simulink model "Sub3_2023"  (R2023b)
settings: Solver=FixedStepDiscrete  StartTime=0.0  StopTime=4.5  FixedStep=75e-6  RelTol=1e-3  EnableMultiTasking=on
undefined symbols (not defined in the file or in its folder): D1, D11, Delta
libraries: spsSeriesRLCBranchLib x41, spsLoadFlowBusLib x29, spsDistributedParametersLineLib x19, spsThreePhaseSeriesRLCLoadLib x15, spsThreePhaseTransformerTwoWindingsLib x13, spsThreePhaseParallelRLCLoadLib x11, spsThreePhaseVIMeasurementLib x11, spsSynchronousMachinepuStandardLib x7, spsExcitationSystemLib x7, spsHydraulicTurbineandGovernorLib x7, spsGenericPowerSystemStabilizerLib x7, spsMultiBandPowerSystemStabilizerLib x7
(part 1 of 5)
settings Model: Creator=The MathWorks, Inc.  LastModifiedBy=dilu2
settings SolverCC: AlgebraicLoopSolver=TrustRegion
settings DataIOCC: SaveFormat=StructureWithTime  SaveOutput=off  SignalLogging=off  DSMLogging=off  SaveTime=off  ReturnWorkspaceOutputs=off
settings OptimizationCC: ExpressionDepthLimit=2147483647  LifeSpan=inf
settings DebuggingCC: UnderspecifiedInitializationDetection=Classic  MergeDetectMultiDrivingBlocksExec=none  SolverPrmCheckMsg=warning  FcnCallInpInsideContextMsg=warning  UnconnectedInputMsg=warning  UnconnectedOutputMsg=warning  UnconnectedLineMsg=warning  StateNameClashWarn=warning  SFUnexpectedBacktrackingDiag=warning  SFNoUnconditionalDefaultTransitionDiag=warning  SFExecutionAtInitializationDiag=none  ArithmeticOperatorsInVariantConditions=warning
settings HardwareCC: ProdBitPerPointer=32  ProdBitPerSizeT=32  ProdBitPerPtrDiffT=32  ProdLargestAtomicFloat=None  ProdIntDivRoundTo=Undefined  ProdEndianess=Unspecified  ProdWordSize=32  ProdHWDeviceType=32-bit Generic
settings ModelReferenceCC: EnableRefExpFcnMdlSchedulingChecks=on  PropagateSignalLabelsOutOfModel=off
settings SFSimCC: SimUseLocalCustomCode=off  CustomCodeUndefinedFunction=UseInterfaceOnly
settings RTWCC: RTWUseLocalCustomCode=off
settings CodeAppCC: StateflowObjectComments=on
settings GRTTargetCC: TargetLangStandard=C89/C90 (ANSI)  CombineOutputUpdateFcns=off  GRTInterface=on
settings ConfigComp: CovMetricSettings=dw  CovSaveCumulativeToWorkspaceVar=on  CovSaveSingleToWorkspaceVar=on  CovExternalEMLEnable=off  CovSFcnEnable=off
settings SimscapeCC: SimscapeNormalizeSystem=off

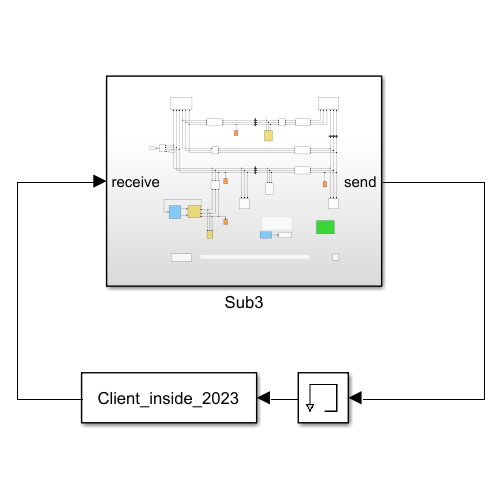
[thumbnail: Simulink's stored preview of the top-level diagram]
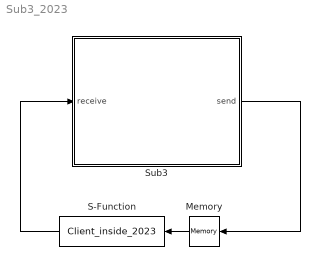
== system Sub3_2023 ==
  Memory : Memory
  S-Function : S-Function  FunctionName=Client_inside_2023  SFunctionDeploymentMode=off  EnableBusSupport=off
  Sub3 : Subsystem
  wires:
  Memory/1 -> S-Function/1
  S-Function/1 -> Sub3/1(receive)
  Sub3/1(send) -> Memory/1

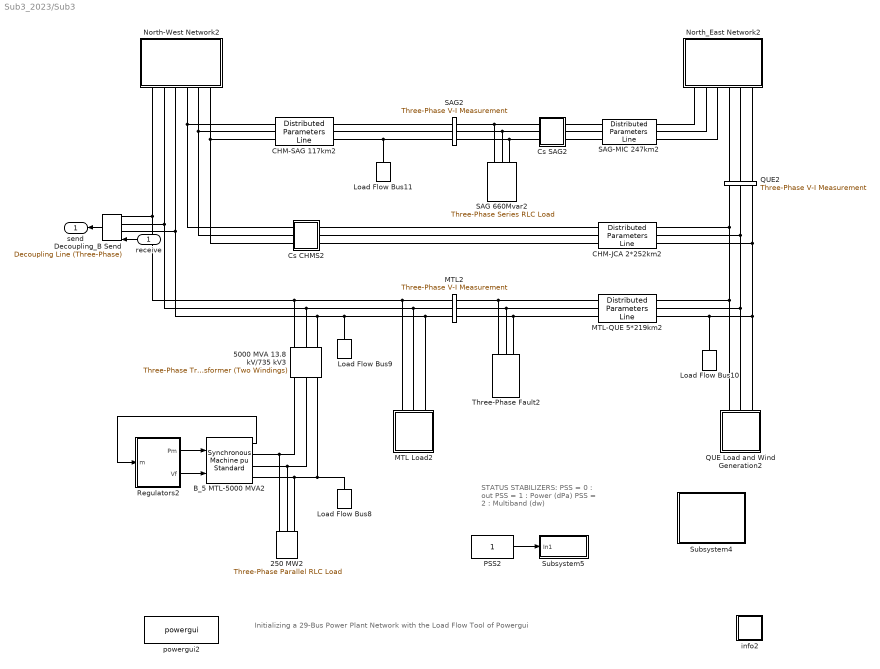
== system Sub3_2023/Sub3 ==
  note: Initializing a 29-Bus Power Plant Network with the Load Flow Tool of Powergui
  note: STATUS STABILIZERS:
      | PSS = 0 :  out
      | PSS = 1 :  Power (dPa)
      | PSS = 2 :  Multiband (dw)
  receive : Inport
  250 MW2 : spsThreePhaseParallelRLCLoadLib/Three-Phase Parallel RLC Load  LConnTagsString=A|B|C  Configuration=Y (grounded)  NominalVoltage=(13800)*1  Vabc=[1e3 1e3 1e3]  Vabcp=[1e3 1e3 1e3]  NominalFrequency=60  UnbalancedPower=off  ActivePower=250000000  InductivePower=0  CapacitivePower=0  Pabc=[10e3 9e3 11e3]  QLabc=[100 90 110]  QCabc=[100 90 110]  Pabcp=[10e3 9e3 11e3]  QLabcp=[100 90 110]  QCabcp=[100 90 110]  Measurements=None  LoadType=constant PQ
  5000 MVA 13.8 kV/735 kV3 : spsThreePhaseTransformerTwoWindingsLib/Three-Phase Transformer (Two Windings)  Winding1Connection=Delta (D1)  Winding2Connection=Yg  CoreType=Three single-phase transformers  SetSaturation=off  Hysteresis=off  DataFile='basic_model'  SetInitialFlux=off  Measurements=None  UNITS=pu  NominalPower=[ 5000e6 60 ]  Winding1="[ 13.8e3 0.002  0.0]"  Winding2=[ 735e3 0.002 0.12]  Rm=500  Lm=500  L0=0.5  Saturation="[ 0,0  ;  0.005,1.2  ;  1.0,1.4 ]"  InitialFluxes=[ 0.8 , -0.8 , 0.7 ]  BreakLoop=off  DiscreteSolver=Trapezoidal iterative  DataType=off  TransfoNumber=0
  B_5 MTL-5000 MVA2 : spsSynchronousMachinepuStandardLib/Synchronous Machine pu Standard  PresetModel=No  MechanicalLoad=Mechanical power Pm  ShowDetailedParameters=on  RotorType=Salient-pole  Units=per unit standard parameters  MeasurementBus=off  NominalParameters="[5000E6  13800   60 ]"  Reactances1=[ 31 32 33 34 35 36 37 ]  Reactances2=[ 1.305, 0.296, 0.252, 0.474, 0.243, 0.18 ]  dAxisTimeConstants=Short-circuit  qAxisTimeConstants=Open-circuit  TimeConstants1=[]  TimeConstants2=[]  TimeConstants3=[]  TimeConstants4=[]  TimeConstants5=[ 1.01, 0.053, 0.1 ]  TimeConstants6=[]  TimeConstants7=[]  TimeConstants8=[]  StatorResistance=2.8544e-3  Mechanical="[ 3.7 0  32]"  PolePairs=32  InitialConditions=[0 -113.876 0.904539 0.904539 0.904539 -42.1129 -162.113 77.8871 1.28555]  SetSaturation=off  Saturation=[0.6404,0.7127,0.8441,0.9214,0.9956,1.082,1.19,1.316,1.457;0.7,0.7698,0.8872,0.9466,0.9969,1.046,1.1,1.151,1.201]  LoadFlowParameters=[1 4000000000 0 0 0]  TsPowergui=0  TsBlock=-1  IterativeModel=Trapezoidal non iterative  IterativeDiscreteModel=Trapezoidal non iterative  BusType=PV  Pref=4500000000  Qref=0  Qmin=-Inf  Qmax=Inf  PLF=0  QLF=0
  CHM-JCA 2*252km2 : spsDistributedParametersLineLib/Distributed Parameters Line  Phases=3  Length=252  Frequency=60  Resistance="[0.01273  0.3864]/2"  Inductance="[0.9337e-3  4.1264e-3]/2"  Capacitance=[12.74e-9 7.751e-9]*2  x1=[-0.0015 2.14788825310089e-08 -52695.4931206876 -817990.561269633;-0.001425 2.14931441848027e-08 -29549.3766894674 -819153.330536621;-0.00135 2.14902245479913e-08 -6379.63893864228 -819661.281164644;-0.001275 2.14701259544877e-08 16795.1985979387 -819514.007105742;-0.0012 2.14328644708e-08 39956.6103097356 -818711.626088545;-0.001125 2.13784698831882e-08 63086.0813186075 -817254.77952416;-0.00105 2.13069856738533e-08 86165.1222793228 -815144.631993441;-0.000975 2.12184689861786e-08 109175.284159659 -812382.870316038;-0.0009 2.11129905790498e-08 132098.172988275 -808971.702201979;-0.000825 2.09906347702916e-08 154915.464558574 -804913.854486862;-0.00075 2.08514993692656e-08 177608.919076792 -800212.570952063;-0.000675 2.06956955986824e-08 200160.395742607 -794871.609731707;-0.0006 2.05233480056924e-08 222551.867250622 -788895.240308476;-0.000525 2.03345943623244e-08 244765.434201114 -782288.240100644;-0.00045 2.01295855553529e-08 266783.339408543 -775055.890643087;-0.000375 1.99084854656814e-08 288587.982096371 -767203.973365303;-0.0003 1.96714708373387e-08 310161.931966855 -758738.764969824;-0.000225 1.94187311361923e-08 331487.943134562 -749667.032414722;-0.00015 1.91504683984921e-08 352548.967912462 -739996.027504197;-7.5e-05 1.88668970693661e-08 373328.170439593 -729733.481091605]  x2=[-0.0015 1.43547805261935e-08 -269861.286315616 -765335.489949611;-0.001425 1.43176491173949e-08 -248116.944399225 -772658.724453944;-0.00135 1.42690723989592e-08 -226174.261593797 -779364.307396023;-0.001275 1.4209089202372e-08 -204050.778544234 -785446.878435444;-0.0012 1.41377474772827e-08 -181764.180424385 -790901.575257983;-0.001125 1.40551042531748e-08 -159332.282799789 -795724.037462462;-0.00105 1.39612255937773e-08 -136773.017386189 -799910.410046378;-0.000975 1.3856186544254e-08 -114104.417715188 -803457.346487544;-0.0009 1.3740071071214e-08 -91344.604718521 -806362.011419237;-0.000825 1.36129719955899e-08 -68511.7722424616 -808622.082896754;-0.00075 1.34749909184379e-08 -45624.1725039369 -810235.754253535;-0.000675 1.33262381397199e-08 -22700.1014999858 -811201.73554539;-0.0006 1.31668325701314e-08 242.115617781237 -811519.254581652;-0.000525 1.29969016360456e-08 23184.1391920279 -811188.057542463;-0.00045 1.28165811776512e-08 46107.6297201337 -810208.409181668;-0.000375 1.26260153403637e-08 68994.2625145116 -808581.092615177;-0.0003 1.24253564595976e-08 91825.742351083 -806307.408694955;-0.000225 1.2214764938992e-08 114583.8180942 -803389.17496914;-0.00015 1.19944091221863e-08 137250.297286324 -799828.72422912;-7.5e-05 1.1764465158249e-08 159807.060690796 -795628.902644742]  x3=[-0.0015 5.32909393588854e-11 -353.825063947876 -933.331217282833;-0.001425 5.27444551797059e-11 -327.297425889231 -942.960561676809;-0.00135 5.2155807890073e-11 -300.508151276149 -951.836117825561;-0.001275 5.15254680456233e-11 -273.478655044866 -959.950790745304;-0.0012 5.08539395303841e-11 -246.230544161103 -967.298093690665;-0.001125 5.01417591539757e-11 -218.785600347792 -973.872153340087;-0.00105 4.93894962224943e-11 -191.165762673095 -979.667714490872;-0.000975 4.85977520834172e-11 -163.393110012651 -984.680144260112;-0.0009 4.77671596448951e-11 -135.489843400061 -988.905435788142;-0.000825 4.6898382869815e-11 -107.478268279722 -992.340211441564;-0.00075 4.59921162450381e-11 -79.3807766761923 -994.981725513273;-0.000675 4.50490842262379e-11 -51.2198292943543 -996.827866417338;-0.0006 4.40700406587813e-11 -23.0179375646682 -997.877158376967;-0.000525 4.30557681751163e-11 5.20235435212098 -998.128762604222;-0.00045 4.20070775691475e-11 33.4184875864397 -997.582477970533;-0.000375 4.09248071480997e-11 61.6079065931019 -996.238741167479;-0.0003 3.98098220623883e-11 89.7480771818661 -994.098626357699;-0.000225 3.8663013614031e-11 117.816504530923 -991.163844316227;-0.00015 3.74852985441545e-11 145.79075116891 -987.436741062925;-7.5e-05 3.62776183001661e-11 173.648454911087 -982.920295987105]  x4=[-0.0015 3.56468616185308e-11 -3930.11452440296 -10267.8671256367;-0.001425 3.68276356651575e-11 -3638.26562484361 -10374.8700196272;-0.00135 3.79789702633153e-11 -3343.50835141109 -10473.5794012647;-0.001275 3.90999450537422e-11 -3046.07832855985 -10563.9163637801;-0.0012 4.01896639463424e-11 -2746.21331729932 -10645.8086931875;-0.001125 4.12472558365064e-11 -2444.15302513141 -10719.190926012;-0.00105 4.22718753014589e-11 -2140.138914432 -10784.0044016194;-0.000975 4.32627032760768e-11 -1834.41400942963 -10840.1973091089;-0.0009 4.42189477076373e-11 -1527.22270193559 -10887.72472873;-0.000825 4.51398441889729e-11 -1218.81055598091 -10926.5486677908;-0.00075 4.60246565695266e-11 -909.424111516214 -10956.6380910284;-0.000675 4.68726775438196e-11 -599.310687331423 -10977.9689454182;-0.0006 4.768322921686e-11 -288.718183352941 -10990.5241794015;-0.000525 4.84556636460423e-11 22.1051175237762 -10994.2937565166;-0.00045 4.91893633591025e-11 332.910747907765 -10989.274663421;-0.000375 4.98837418477159e-11 643.450254533582 -10975.470912301;-0.0003 5.05382440363431e-11 953.475396871044 -10952.893537664;-0.000225 5.11523467259487e-11 1262.73834556491 -10921.5605875179;-0.00015 5.17255590122387e-11 1570.99188054588 -10881.4971089437;-7.5e-05 5.2257422678082e-11 1877.98958865452 -10832.735128073]  x5=0.00142516474882927  V1=ones(3,3)  V2=ones(3,3)  I1=ones(3,3)  I2=ones(3,3)  nHarmo=1  Measurements=None  Decoupling=on  VsMag0=[669271.096488228 669270.652926469 669270.90062472]  VrMag0=[662602.894278608 662603.037872478 662602.726163221]  VsAngle0=[-1.28592943401852 -121.285926872022 118.714104732553]  VrAngle0=[-17.0228975012821 -137.022921456009 102.977079768198]  IsMag0=[819.838115462759 819.831333521817 819.822841412156]  IrMag0=[9030.15416595123 9030.15837069581 9030.1660687479]  IsAngle0=[-18.3607604375241 -138.36171938416 101.639170566658]  IrAngle0=[-18.5448447465942 -138.544772943748 101.455168050306]
      settings: AttributesFormatString=\n  LibrarySourceBlock=sps_lib/Power Grid Elements/Distributed Parameters Line
  CHM-SAG 117km2 : spsDistributedParametersLineLib/Distributed Parameters Line  Phases=3  Length=117  Frequency=60  Resistance="[0.01273  0.3864]"  Inductance="[0.9337e-3  4.1264e-3]"  Capacitance=[12.74e-9 7.751e-9]  x1=[-0.000675 1.98658437347204e-08 120099.384212573 -820048.654169142;-0.0006 1.97055789462812e-08 143234.627617142 -816325.600270959;-0.000525 1.95295618195378e-08 166255.371451958 -811949.988178119;-0.00045 1.93379330598881e-08 189143.213286628 -806925.315687981;-0.000375 1.91308458524307e-08 211879.856930585 -801255.599446853;-0.0003 1.89084657395106e-08 234447.127058782 -794945.37173915;-0.000225 1.86709704883876e-08 256826.983740769 -787999.67686435;-0.00015 1.84185499491316e-08 279001.536861539 -780424.067104664;-7.5e-05 1.81514059028595e-08 300953.060422608 -772224.598286623]  x2=[-0.000675 1.36464150047778e-08 166130.546631654 -803426.098272825;-0.0006 1.3510914913813e-08 188777.466023371 -798408.377649309;-0.000525 1.33646144041902e-08 211273.479597141 -792752.421584757;-0.00045 1.3207630426298e-08 233600.604383914 -786462.751363909;-0.000375 1.30400884707266e-08 255740.992421751 -779544.394852905;-0.0003 1.28621224679518e-08 277676.945023215 -772002.882480085;-0.000225 1.26738746812731e-08 299390.926923427 -763844.24281505;-0.00015 1.2475495593091e-08 320865.580297491 -755074.997749517;-7.5e-05 1.22671437846133e-08 342083.738636073 -745702.157283819]  x3=[-0.000675 1.56671377221203e-11 655.342290944049 -4153.32595111528;-0.0006 1.47007289951298e-11 772.497655199839 -4133.1388980955;-0.000525 1.37225687303092e-11 889.035496649674 -4109.64787707972;-0.00045 1.2733438854008e-11 1004.86265672619 -4082.87166643073;-0.000375 1.1734130061515e-11 1119.88654496983 -4052.83167064162;-0.0003 1.07254411849891e-11 1234.01521304425 -4019.55190322541;-0.000225 9.70817855488465e-12 1347.15742823844 -3983.05896751897;-0.00015 8.68315535538353e-12 1459.2227463967 -3943.38203541674;-7.5e-05 7.65119097434806e-12 1570.12158421834 -3900.55282405116]  x4=[-0.000675 2.87955679117454e-11 -58.179032260622 -1899.1904056796;-0.0006 2.95286509391463e-11 -4.4649544291961 -1900.07615984008;-0.000525 3.02381292147899e-11 49.2526926184844 -1899.44302219052;-0.00045 3.0923435592598e-11 102.930967817277 -1897.29149885148;-0.000375 3.15840222491379e-11 156.526961575294 -1893.62330971778;-0.0003 3.22193611215436e-11 209.99783007517 -1888.44138708371;-0.000225 3.28289443296414e-11 263.300829522758 -1881.74987329893;-0.00015 3.34122845819419e-11 316.393350315863 -1873.55411745716;-7.5e-05 3.39689155651726e-11 369.232951105707 -1863.86067112024]  x5=0.000661683633385019  V1=ones(3,3)  V2=ones(3,3)  I1=ones(3,3)  I2=ones(3,3)  nHarmo=1  Measurements=None  Decoupling=on  VsMag0=[676709.77841619 676709.532429466 676709.555770503]  VrMag0=[669872.175479888 669872.308250308 669872.011404575]  VsAngle0=[-7.08802978836752 -127.088039531023 112.911983377236]  VrAngle0=[-3.73716141990226 -123.737184181178 116.262817364722]  IsMag0=[3442.59994794228 3442.59576511442 3442.58917191232]  IrMag0=[1555.67453781717 1555.67655932668 1555.6835352225]  IsAngle0=[-6.45330477220459 -126.453471672169 113.546672066862]  IrAngle0=[-17.1748303043255 -137.174490649355 102.825275045827]
      settings: AttributesFormatString=\n  LibrarySourceBlock=sps_lib/Power Grid Elements/Distributed Parameters Line
  Cs CHMS2 : Subsystem  mask{Xc=33/2}
      mask prompts: Xc "Condensator Reactance at  60Hz  (ohm):"
      mask help: Series Compensation
      mask init:
      | Cs=1/Xc/(2*pi*60);
      mask Display: disp('Cs')
  Cs SAG2 : Subsystem  mask{Xc=22}
      mask prompts: Xc "Condensator Reactance at  60Hz  (ohm):"
      mask help: Series Compensation
      mask init:
      | Cs=1/Xc/(2*pi*60);
      mask Display: disp('Cs')
  Decoupling_B Send : spsDecouplingLineThreePhaseLib/Decoupling Line (Three-Phase)  Length=252  Frequency=60  Resistance="[0.01273  0.3864]/2"  Inductance="[0.9337e-3  4.1264e-3]/2"  Capacitance=[12.74e-9 7.751e-9]*2  VsMag0=[645716.873803131 645717.117585077 645717.103800347]  VsAngle0=[95.8608940156624 -144.139117060793 -24.1390927893461]  IhsMag0=[6636.13895491375 6636.14647590145 6636.14203567859]  IhsAngle0=[111.871942870248 -128.128050353118 -8.12799750568943]  ShowPorts=on  ConnectorID=T42_4043_2846767750151_S
      settings: LibrarySourceBlock=|
      | sps_lib/Power Grid Elements/Decoupling Line
      | (Three-Phase)
  Load Flow Bus10 : spsLoadFlowBusLib/Load Flow Bus  LConnTagsString=a  Phases=single  Connectors=on one side  ID=QUE7  Vbase=735e3  Vref=1  Vangle=0  VLF=1.023  VLFb=1  VLFc=1  angleLF=-14.99  angleLFb=0  angleLFc=0
      settings: AttributesFormatString=%<ID>\n%<Vbase>V\n%<VLF>pu\n%<angleLF>deg.
  Load Flow Bus11 : spsLoadFlowBusLib/Load Flow Bus  LConnTagsString=a  Phases=single  Connectors=on one side  ID=SAG7  Vbase=735e3  Vref=1  Vangle=0  VLF=1.036  VLFb=1  VLFc=1  angleLF=-0.1653  angleLFb=0  angleLFc=0
      settings: AttributesFormatString=%<ID>\n%<Vbase>V\n%<VLF>pu\n%<angleLF>deg.
  Load Flow Bus8 : spsLoadFlowBusLib/Load Flow Bus  LConnTagsString=a  Phases=single  Connectors=on one side  ID=MTL_13.8  Vbase=13.8e3  Vref=1  Vangle=0  VLF=1  VLFb=1  VLFc=1  angleLF=-47.86  angleLFb=0  angleLFc=0
      settings: AttributesFormatString=%<ID>\n%<Vbase>V\n%<VLF>pu\n%<angleLF>deg.
  Load Flow Bus9 : spsLoadFlowBusLib/Load Flow Bus  LConnTagsString=a  Phases=single  Connectors=on one side  ID=MTL7  Vbase=735e3  Vref=1  Vangle=0  VLF=1.013  VLFb=1  VLFc=1  angleLF=-23.64  angleLFb=0  angleLFc=0
      settings: AttributesFormatString=%<ID>\n%<Vbase>V\n%<VLF>pu\n%<angleLF>deg.
  MTL Load2 : Subsystem
  MTL-QUE 5*219km2 : spsDistributedParametersLineLib/Distributed Parameters Line  Phases=3  Length=219  Frequency=60  Resistance="[0.01273  0.3864]/5"  Inductance="[0.9337e-3  4.1264e-3]/5"  Capacitance=[12.74e-9 7.751e-9]*5  x1=[-0.001275 8.97642211389418e-08 0 0;-0.0012 8.97304952684457e-08 0 0;-0.001125 8.96250402129547e-08 0 0;-0.00105 8.94479402716265e-08 0 0;-0.000975 8.91993370154446e-08 0 0;-0.0009 8.88794291740481e-08 0 0;-0.000825 8.84884724768708e-08 -163872.459638605 -773673.870997315;-0.00075 8.80267794487145e-08 -141934.751428708 -777997.40505494;-0.000675 8.74947191599218e-08 -119883.582750192 -781699.019890724;-0.0006 8.68927169313467e-08 -97736.5809699071 -784775.756490403;-0.000525 8.62212539943599e-08 -75511.4500622143 -787225.155357816;-0.00045 8.54808671061594e-08 -53225.9564567056 -789045.258480985;-0.000375 8.46721481206953e-08 -30897.9148359899 -790234.610897321;-0.0003 8.37957435155509e-08 -8545.17389490828 -790792.261856701;-0.000225 8.28523538751581e-08 13814.3979274394 -790717.765581479;-0.00015 8.18427333307609e-08 36162.9267314513 -790011.18162284;-7.5e-05 8.0767688957575e-08 58482.5474451453 -788673.074813188]  x2=[-0.001275 1.4209089202372e-08 0 0;-0.0012 1.41377474772827e-08 0 0;-0.001125 1.40551042531748e-08 0 0;-0.00105 1.39612255937773e-08 0 0;-0.000975 1.3856186544254e-08 0 0;-0.0009 1.3740071071214e-08 0 0;-0.000825 1.36129719955899e-08 -68511.7722424616 -808622.082896754;-0.00075 1.34749909184379e-08 -45624.1725039369 -810235.754253535;-0.000675 1.33262381397199e-08 -22700.1014999858 -811201.73554539;-0.0006 1.31668325701314e-08 242.115617781237 -811519.254581652;-0.000525 1.29969016360456e-08 23184.1391920279 -811188.057542463;-0.00045 1.28165811776512e-08 46107.6297201337 -810208.409181668;-0.000375 1.26260153403637e-08 68994.2625145116 -808581.092615177;-0.0003 1.24253564595976e-08 91825.742351083 -806307.408694955;-0.000225 1.2214764938992e-08 114583.8180942 -803389.17496914;-0.00015 1.19944091221863e-08 137250.297286324 -799828.72422912;-7.5e-05 1.1764465158249e-08 159807.060690796 -795628.902644742]  x3=[-0.001275 3.55264360188674e-10 0 0;-0.0012 3.29669675506793e-10 0 0;-0.001125 3.03811457930428e-10 0 0;-0.00105 2.77710378123064e-10 0 0;-0.000975 2.5138730088854e-10 0 0;-0.0009 2.2486326849204e-10 0 0;-0.000825 1.98159483839231e-10 -7102.47823834771 -20057.5471743782;-0.00075 1.71297293526982e-10 -6532.60058481189 -20250.3213202449;-0.000675 1.44298170779225e-10 -5957.5008703207 -20426.9076690885;-0.0006 1.17183698281583e-10 -5377.63882078661 -20587.1650604835;-0.000525 8.99755509285052e-11 -4793.47796905981 -20730.9653871235;-0.00045 6.26954784966872e-11 -4205.48528438722 -20858.1936972273;-0.000375 3.53652882586321e-11 -3614.13079912437 -20968.7482864307;-0.0003 8.00682755025e-12 -3019.88723299875 -21062.5407790865;-0.000225 -1.93580336935672e-11 -2423.22961522491 -21139.4961989112;-0.00015 -4.67074204214376e-11 -1824.6349047733 -21199.5530289196;-7.5e-05 -7.40194699520705e-11 -1224.58160909667 -21242.6632606007]  x4=[-0.001275 2.99597844132757e-10 0 0;-0.0012 3.28836590243948e-10 0 0;-0.001125 3.57812469416266e-10 0 0;-0.00105 3.86502318775247e-10 0 0;-0.000975 4.14883204094284e-10 0 0;-0.0009 4.42932438127893e-10 0 0;-0.000825 4.70627598747556e-10 -1323.85659522413 -8328.03394763917;-0.00075 4.97946546865624e-10 -1087.88942341492 -8362.13156092163;-0.000675 5.24867444132966e-10 -851.052609445902 -8389.54461417919;-0.0006 5.51368770396209e-10 -613.535477042433 -8410.25119383652;-0.000525 5.77429340900622e-10 -375.527893766024 -8424.23474737065;-0.00045 6.03028323224884e-10 -137.220119237107 -8431.48409654284;-0.000375 6.28145253934203e-10 101.197346955589 -8431.9934463343;-0.0003 6.52760054938472e-10 339.5339175375 -8425.76238957858;-0.000225 6.76853049542387e-10 577.599069900775 -8412.79590728711;-0.00015 7.00404978174696e-10 815.202498405133 -8393.10436466746;-7.5e-05 7.23397013784009e-10 1052.15426650528 -8366.70350283749]  x5=0.00123853603172068  V1=ones(3,3)  V2=ones(3,3)  I1=ones(3,3)  I2=ones(3,3)  nHarmo=1  Measurements=None  Decoupling=on  VsMag0=[645717.103800377 645717.117585074 645716.873803133]  VrMag0=[662602.894278608 662603.037872478 662602.726163221]  VsAngle0=[-24.1390927893337 -144.139117060795 95.8608940156664]  VrAngle0=[-17.0228975012821 -137.022921456009 102.977079768198]  IsMag0=[17463.0562889059 17463.0593352233 17463.044410006]  IrMag0=[6920.72764335611 6920.72903749753 6920.73301494449]  IsAngle0=[-31.6792680234145 -151.679318797623 88.3206979336596]  IrAngle0=[-21.2124174849752 -141.212372798414 98.7875948627143]
      settings: AttributesFormatString=\n  LibrarySourceBlock=sps_lib/Power Grid Elements/Distributed Parameters Line
  MTL2 : spsThreePhaseVIMeasurementLib/Three-Phase V-I Measurement  VoltageMeasurement=phase-to-ground  SetLabelV=on  LabelV=Vabc_MTL7_2  Vpu=on  VpuLL=off  CurrentMeasurement=no  SetLabelI=off  LabelI=A1  Ipu=off  Pbase=100e6  Vbase=735e3  OutputType=Magnitude  PhasorSimulation=off  PSBequivalent=0
  North-West Network2 : Subsystem
  North_East Network2 : Subsystem
  PSS2 : Constant
  QUE Load and Wind Generation2 : Subsystem
  QUE2 : spsThreePhaseVIMeasurementLib/Three-Phase V-I Measurement  VoltageMeasurement=no  SetLabelV=on  LabelV=Vabc_QUE7  Vpu=on  VpuLL=off  CurrentMeasurement=no  SetLabelI=off  LabelI=A1  Ipu=off  Pbase=100e6  Vbase=735e3  OutputType=Magnitude  PhasorSimulation=off  PSBequivalent=0
  Regulators2 : Subsystem
  SAG 660Mvar2 : spsThreePhaseSeriesRLCLoadLib/Three-Phase Series RLC Load  LConnTagsString=A|B|C  Configuration=Y (grounded)  NominalVoltage=735e3  Vabc=[1e3 1e3 1e3]  Vabcp=[1e3 1e3 1e3]  NominalFrequency=60  UnbalancedPower=off  ActivePower=2200000  InductivePower=660e6  CapacitivePower=0  Pabc=[10e3 9e3 11e3]  QLabc=[100 90 110]  QCabc=[100 90 110]  Pabcp=[10e3 9e3 11e3]  QLabcp=[100 90 110]  QCabcp=[100 90 110]  Measurements=None  LoadType=constant Z
  SAG-MIC 247km2 : spsDistributedParametersLineLib/Distributed Parameters Line  Phases=3  Length=247  Frequency=60  Resistance="[0.01273  0.3864]/1"  Inductance="[0.9337e-3  4.1264e-3]/1"  Capacitance=[12.74e-9 7.751e-9]*1  x1=[-0.001425 1.51965491715446e-08 -89449.2345900926 -803563.355726872;-0.00135 1.5173434542913e-08 -66696.2840151997 -805770.954430085;-0.001275 1.51381905028692e-08 -43890.0174513524 -807334.432161035;-0.0012 1.50908452249594e-08 -21048.6658790944 -808252.539099548;-0.001125 1.50314365562744e-08 1809.511674612 -808524.541324982;-0.00105 1.49600119871951e-08 24666.2427323723 -808150.221402922;-0.000975 1.48766286134291e-08 47503.2559730984 -807129.878558985;-0.0009 1.47813530903695e-08 70302.2958378238 -805464.328439629;-0.000825 1.46742615798118e-08 93045.1371229176 -803154.902460136;-0.00075 1.4555439689071e-08 115713.599549034 -800203.446740299;-0.000675 1.44249824025483e-08 138289.562294148 -796612.320628661;-0.0006 1.42829940058027e-08 160754.978479065 -792384.394816489;-0.000525 1.4129588002186e-08 183091.88959382 -787523.049042989;-0.00045 1.39648870221104e-08 205282.439853433 -782032.169393591;-0.000375 1.37890227250191e-08 227308.890471555 -775916.145193473;-0.0003 1.36021356941406e-08 249153.633840576 -769179.865498802;-0.000225 1.34043753241079e-08 270799.207606883 -761828.715188499;-0.00015 1.31958997015349e-08 292228.308629996 -753868.570659643;-7.5e-05 1.29768754786445e-08 313423.806814433 -745305.795129979]  x2=[-0.001425 4.80264229603194e-09 11099.4849218779 -821643.782393996;-0.00135 4.76571614242728e-09 34323.4076602216 -821001.616626406;-0.001275 4.72498034825626e-09 57519.8927916473 -819703.15472823;-0.0012 4.68046747708947e-09 80670.3974008593 -817749.434670043;-0.001125 4.63221311183505e-09 103756.415328688 -815142.018225766;-0.00105 4.58025582629427e-09 126759.491965629 -811882.989724212;-0.000975 4.52463715432621e-09 149661.239004177 -807974.954382897;-0.0009 4.46540155664625e-09 172443.34913816 -803421.036225481;-0.000825 4.40259638528484e-09 195087.610697313 -798224.87558446;-0.00075 4.33627184573503e-09 217575.922205416 -792390.626191147;-0.000675 4.26648095681891e-09 239890.30685033 -785922.95185524;-0.0006 4.19327950830526e-09 262012.926854394 -778827.022736644;-0.000525 4.116726016312e-09 283926.097733662 -771108.511212526;-0.00045 4.03688167652932e-09 305612.302434616 -762773.5873429;-0.000375 3.95381031530078e-09 327054.20533703 -753828.913938379;-0.0003 3.86757833860152e-09 348234.666111794 -744281.641234026;-0.000225 3.77825467895431e-09 369136.753422638 -734139.401173561;-0.00015 3.68591074032598e-09 389743.758460777 -723410.301308507;-7.5e-05 3.59062034104816e-09 410039.208301682 -712102.918317136]  x3=[-0.001425 1.53482070239555e-11 -974.267486517461 -4064.8150690785;-0.00135 1.47665670520247e-11 -858.963058340455 -4090.73328748301;-0.001275 1.41731229123285e-11 -742.971988237187 -4113.38143628781;-0.0012 1.35683489950324e-11 -626.386997694374 -4132.7414109093;-0.001125 1.29527287471522e-11 -509.301282969648 -4148.79773527997;-0.00105 1.2326754286095e-11 -391.808440591886 -4161.53757421979;-0.000975 1.16909260062672e-11 -274.002392541585 -4170.95074369644;-0.0009 1.10457521790671e-11 -155.977311171064 -4177.02971896627;-0.000825 1.03917485465808e-11 -37.8275439245253 -4179.76964058945;-0.00075 9.72943790930539e-12 80.3524620818455 -4179.16831831456;-0.000675 9.05934970823069e-12 198.468235559462 -4175.22623282944;-0.0006 8.38201960161192e-12 316.425356566239 -4167.94653537689;-0.000525 7.69798903677283e-12 434.129531984446 -4157.33504523568;-0.00045 7.00780481728092e-12 551.48667089719 -4143.40024506867;-0.000375 6.31201866584109e-12 668.402959803247 -4126.15327414191;-0.0003 5.6111867832569e-12 784.784937610146 -4105.60791942005;-0.000225 4.90586940381222e-12 900.539570345532 -4081.78060454532;-0.00015 4.19663034742845e-12 1015.5743255271 -4054.69037670865;-7.5e-05 3.48403656895555e-12 1129.79724613165 -4024.35889142369]  x4=[-0.001425 1.20697872634544e-11 -279.355223170463 -1839.3774898857;-0.00135 1.27745410723097e-11 -227.243591664026 -1846.54010495167;-0.001275 1.34690831084889e-11 -174.950305107357 -1852.22662411075;-0.0012 1.4152858165715e-11 -122.517165953615 -1856.43250164654;-0.001125 1.48253196446694e-11 -69.9860884519846 -1859.15437544488;-0.00105 1.54859299899349e-11 -17.399065142069 -1860.3900696815;-0.000975 1.61341611197091e-11 35.2018667143068 -1860.13859656134;-0.0009 1.67694948479452e-11 87.7746587370375 -1858.40015710817;-0.000825 1.73914232985816e-11 140.277285040571 -1855.17614100388;-0.00075 1.79994493115309e-11 192.667775828758 -1850.46912547762;-0.000675 1.85930868401014e-11 244.904250944863 -1844.28287324558;-0.0006 1.91718613395356e-11 296.944953349924 -1836.62232950314;-0.000525 1.97353101463544e-11 348.748282502686 -1827.49361797176;-0.00045 2.02829828482025e-11 400.272827614444 -1816.90403600377;-0.000375 2.08144416439018e-11 451.477400752186 -1804.86204874895;-0.0003 2.13292616934226e-11 502.321069763603 -1791.37728238768;-0.000225 2.18270314574943e-11 552.763190997621 -1776.46051643587;-0.00015 2.23073530265837e-11 602.763441794316 -1760.12367512797;-7.5e-05 2.27698424389776e-11 652.281852718231 -1742.37981788497]  x5=0.00139688767047948  V1=ones(3,3)  V2=ones(3,3)  I1=ones(3,3)  I2=ones(3,3)  nHarmo=1  Measurements=None  Decoupling=on  VsMag0=[660159.371339391 660159.297704505 660159.177083874]  VrMag0=[670930.718084371 670931.402748966 670930.538861449]  VsAngle0=[-5.57176017470041 -125.571775952741 114.428237470905]  VrAngle0=[1.55396261636306 -118.446088813405 121.553886266144]  IsMag0=[3432.79562093215 3432.79304132191 3432.78494377833]  IrMag0=[1527.90652507594 1527.91221755778 1527.91604324767]  IsAngle0=[-12.6984164906704 -132.698597410847 107.301530336561]  IrAngle0=[-7.85604515006738 -127.855756251268 112.143914434288]
      settings: AttributesFormatString=\n  LibrarySourceBlock=sps_lib/Power Grid Elements/Distributed Parameters Line
  SAG2 : spsThreePhaseVIMeasurementLib/Three-Phase V-I Measurement  VoltageMeasurement=no  SetLabelV=on  LabelV=Vabc_SAG7  Vpu=on  VpuLL=off  CurrentMeasurement=no  SetLabelI=off  LabelI=Iabc_SAG7  Ipu=off  Pbase=100e6  Vbase=735e3  OutputType=Magnitude  PhasorSimulation=off  PSBequivalent=0
  Subsystem4 : Subsystem
      mask Display: disp('Display\nWaveforms')
  Subsystem5 : Subsystem
      mask Display: disp('PSS_select')
  Three-Phase Fault2 : spsThreePhaseFaultLib/Three-Phase Fault  InitialStates=0  FaultA=on  FaultB=on  FaultC=on  GroundFault=on  SwitchTimes=[0.2 0.3]  External=off  SwitchStatus=NaN  FaultResistance=0.001  GroundResistance=0.001  SnubberResistance=1e6  SnubberCapacitance=inf  Measurements=None
  info2 : Subsystem
      settings: OpenFcn="showExample(\"simscapeelectricalsps/LoadFlow29BusNetworkExample\")"
      mask Display: disp('?')
  powergui2 : sps_lib/powergui  Priority=1  SimulationMode=Discrete  SampleTime=75e-6  frequency=60  Iterations=50  frequencyindice=60  Pbase=1e+008  ErrMax=0.0001  UnitsV=kV  UnitsW=MW  buscounter=0  FunctionMessages=off  echomessages=off  EnableUseOfTLC=off  CurrentSourceSwitches=off  DisableSnubberDevices=off  DisableRonSwitches=off  DisableVfSwitches=off  DisplayEquations=off  AutomaticDiscreteSolvers=off  SolverType=Tustin/Backward Euler (TBE)  Interpol=off  ExternalGateDelay=off  methode=off  Ts=100  x0status=blocks  SPID=off  SwTol=0  HookPort=off  NonlinearTolerance=1e-4  nMaxIteration=100  ContinueOnMaxIteration=off  RestoreLinks=warning  ResistiveCurrentMeasurement=off  Frange=[0:2:500]  Ylog=off  Xlog=on  ShowGrid=off  save=off  variable=ZData  structure=0  ZoomFFT=off  StartTime=0.0  cycles=1  DisplayStyle=1  fundamental=60  FreqAxis=off  MaxFrequency=1000  frequencyindicesteady=1  RmsSteady=1  display=off
  send : Outport
  wires:
  Regulators2/2(Vf) -> B_5 MTL-5000 MVA2/2
  B_5 MTL-5000 MVA2/1 -> Regulators2/1(m)
  PSS2/1 -> Subsystem5/1(In1)
  receive/1 -> Decoupling_B Send/1
  Decoupling_B Send/1 -> send/1
  Regulators2/1(Pm) -> B_5 MTL-5000 MVA2/1
  connections:
  Load Flow Bus10/LConn1 -- QUE Load and Wind Generation2/LConn3 -- QUE2/LConn3 -- CHM-JCA 2*252km2/RConn3 -- MTL-QUE 5*219km2/RConn3
  CHM-SAG 117km2/RConn3 -- SAG2/LConn3 -- Load Flow Bus11/LConn1
  5000 MVA 13.8 kV/735 kV3/RConn2 -- Decoupling_B Send/LConn2 -- North-West Network2/RConn2 -- MTL2/LConn2 -- MTL Load2/LConn2
  5000 MVA 13.8 kV/735 kV3/LConn3 -- Load Flow Bus8/LConn1 -- 250 MW2/LConn3 -- B_5 MTL-5000 MVA2/RConn3
  CHM-SAG 117km2/LConn3 -- North-West Network2/RConn6 -- Cs CHMS2/LConn3
  MTL-QUE 5*219km2/LConn3 -- MTL2/RConn3 -- Three-Phase Fault2/LConn3
  MTL Load2/LConn1 -- MTL2/LConn1 -- Decoupling_B Send/LConn3 -- North-West Network2/RConn1 -- 5000 MVA 13.8 kV/735 kV3/RConn1
  Cs CHMS2/RConn3 -- CHM-JCA 2*252km2/LConn3
  MTL-QUE 5*219km2/RConn1 -- QUE Load and Wind Generation2/LConn1 -- QUE2/LConn1 -- CHM-JCA 2*252km2/RConn1
  MTL-QUE 5*219km2/LConn2 -- MTL2/RConn2 -- Three-Phase Fault2/LConn2
  250 MW2/LConn2 -- 5000 MVA 13.8 kV/735 kV3/LConn2 -- B_5 MTL-5000 MVA2/RConn2
  Cs CHMS2/RConn1 -- CHM-JCA 2*252km2/LConn1
  Cs SAG2/RConn3 -- SAG-MIC 247km2/LConn3
  MTL-QUE 5*219km2/RConn2 -- QUE Load and Wind Generation2/LConn2 -- QUE2/LConn2 -- CHM-JCA 2*252km2/RConn2
  Cs SAG2/RConn1 -- SAG-MIC 247km2/LConn1
  QUE2/RConn2 -- North_East Network2/LConn5
  250 MW2/LConn1 -- 5000 MVA 13.8 kV/735 kV3/LConn1 -- B_5 MTL-5000 MVA2/RConn1
  MTL-QUE 5*219km2/LConn1 -- MTL2/RConn1 -- Three-Phase Fault2/LConn1
  QUE2/RConn3 -- North_East Network2/LConn6
  CHM-SAG 117km2/LConn1 -- North-West Network2/RConn4 -- Cs CHMS2/LConn1
  5000 MVA 13.8 kV/735 kV3/RConn3 -- Decoupling_B Send/LConn1 -- North-West Network2/RConn3 -- MTL2/LConn3 -- MTL Load2/LConn3 -- Load Flow Bus9/LConn1
  SAG2/RConn1 -- SAG 660Mvar2/LConn1 -- Cs SAG2/LConn1
  Cs CHMS2/RConn2 -- CHM-JCA 2*252km2/LConn2
  SAG-MIC 247km2/RConn1 -- North_East Network2/LConn1
  SAG-MIC 247km2/RConn3 -- North_East Network2/LConn3
  SAG2/LConn1 -- CHM-SAG 117km2/RConn1
  Cs SAG2/RConn2 -- SAG-MIC 247km2/LConn2
  SAG2/LConn2 -- CHM-SAG 117km2/RConn2
  QUE2/RConn1 -- North_East Network2/LConn4
  SAG2/RConn2 -- SAG 660Mvar2/LConn2 -- Cs SAG2/LConn2
  SAG-MIC 247km2/RConn2 -- North_East Network2/LConn2
  SAG2/RConn3 -- SAG 660Mvar2/LConn3 -- Cs SAG2/LConn3
  CHM-SAG 117km2/LConn2 -- North-West Network2/RConn5 -- Cs CHMS2/LConn2

== system Sub3_2023/Sub3/Cs CHMS2 ==
  note: B
  Ca : spsSeriesRLCBranchLib/Series RLC Branch  LConnTagsString=__new0  RConnTagsString=__new0  BranchType=C  Resistance=1.0  Inductance=1.0  SetiL0=off  InitialCurrent=0  Capacitance=Cs  Setx0=off  InitialVoltage=0  Measurements=None
  Cb : spsSeriesRLCBranchLib/Series RLC Branch  LConnTagsString=__new0  RConnTagsString=__new0  BranchType=C  Resistance=1.0  Inductance=1.0  SetiL0=off  InitialCurrent=0  Capacitance=Cs  Setx0=off  InitialVoltage=0  Measurements=None
  Cc : spsSeriesRLCBranchLib/Series RLC Branch  LConnTagsString=__new0  RConnTagsString=__new0  BranchType=C  Resistance=1.0  Inductance=1.0  SetiL0=off  InitialCurrent=0  Capacitance=Cs  Setx0=off  InitialVoltage=0  Measurements=None
  A : PMIOPort  Side=Left
  B : PMIOPort  Port=2  Side=Left
  C : PMIOPort  Port=3  Side=Left
  "A " : PMIOPort  Port=4  Side=Right
  "B " : PMIOPort  Port=5  Side=Right
  "C " : PMIOPort  Port=6  Side=Right
  connections:
  Cc/RConn1 -- "C "/RConn1
  C/RConn1 -- Cc/LConn1
  Cb/RConn1 -- "B "/RConn1
  B/RConn1 -- Cb/LConn1
  Ca/RConn1 -- "A "/RConn1
  A/RConn1 -- Ca/LConn1

== system Sub3_2023/Sub3/Cs SAG2 ==
  note: B
  Ca : spsSeriesRLCBranchLib/Series RLC Branch  LConnTagsString=__new0  RConnTagsString=__new0  BranchType=C  Resistance=1.0  Inductance=1.0  SetiL0=off  InitialCurrent=0  Capacitance=Cs  Setx0=off  InitialVoltage=0  Measurements=None
  Cb : spsSeriesRLCBranchLib/Series RLC Branch  LConnTagsString=__new0  RConnTagsString=__new0  BranchType=C  Resistance=1.0  Inductance=1.0  SetiL0=off  InitialCurrent=0  Capacitance=Cs  Setx0=off  InitialVoltage=0  Measurements=None
  Cc : spsSeriesRLCBranchLib/Series RLC Branch  LConnTagsString=__new0  RConnTagsString=__new0  BranchType=C  Resistance=1.0  Inductance=1.0  SetiL0=off  InitialCurrent=0  Capacitance=Cs  Setx0=off  InitialVoltage=0  Measurements=None
  A : PMIOPort  Side=Left
  B : PMIOPort  Port=2  Side=Left
  C : PMIOPort  Port=3  Side=Left
  "A " : PMIOPort  Port=4  Side=Right
  "B " : PMIOPort  Port=5  Side=Right
  "C " : PMIOPort  Port=6  Side=Right
  connections:
  A/RConn1 -- Ca/LConn1
  Ca/RConn1 -- "A "/RConn1
  B/RConn1 -- Cb/LConn1
  Cb/RConn1 -- "B "/RConn1
  C/RConn1 -- Cc/LConn1
  Cc/RConn1 -- "C "/RConn1

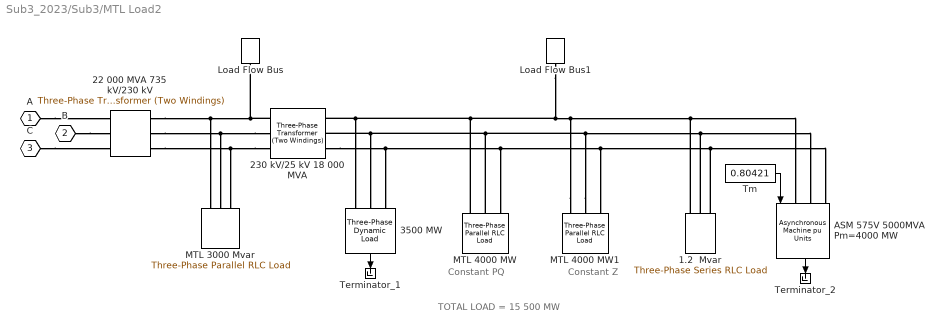
== system Sub3_2023/Sub3/MTL Load2 ==
  note: Constant PQ
  note: Constant Z
  note: TOTAL LOAD = 15 500 MW
  1.2  Mvar : spsThreePhaseSeriesRLCLoadLib/Three-Phase Series RLC Load  LConnTagsString=A|B|C  Configuration=Y (grounded)  NominalVoltage=25e3  Vabc=[1e3 1e3 1e3]  Vabcp=[1e3 1e3 1e3]  NominalFrequency=60  UnbalancedPower=off  ActivePower=2000e6/50  InductivePower=0  CapacitivePower=2000e6  Pabc=[10e3 9e3 11e3]  QLabc=[100 90 110]  QCabc=[100 90 110]  Pabcp=[10e3 9e3 11e3]  QLabcp=[100 90 110]  QCabcp=[100 90 110]  Measurements=None  LoadType=constant Z
  22 000 MVA 735 kV/230 kV : spsThreePhaseTransformerTwoWindingsLib/Three-Phase Transformer (Two Windings)  Winding1Connection=Yg  Winding2Connection=Delta (D1)  CoreType=Three single-phase transformers  SetSaturation=off  Hysteresis=off  DataFile='basic_model'  SetInitialFlux=off  Measurements=None  UNITS=pu  NominalPower=[ 22000e6 60 ]  Winding1="[ 735e3 0.002  0.12]"  Winding2=[230e3 0.002 0]  Rm=500  Lm=500  L0=0.5  Saturation="[ 0,0  ;  0.005,1.2  ;  1.0,1.4 ]"  InitialFluxes=[ 0.8 , -0.8 , 0.7 ]  BreakLoop=off  DiscreteSolver=Trapezoidal iterative  DataType=off  TransfoNumber=0
  230 kV/25 kV 18 000 MVA : spsThreePhaseTransformerTwoWindingsLib/Three-Phase Transformer (Two Windings)  Winding1Connection=Yg  Winding2Connection=Delta (D1)  CoreType=Three single-phase transformers  SetSaturation=off  Hysteresis=off  DataFile='basic_model'  SetInitialFlux=off  Measurements=None  UNITS=pu  NominalPower=[18000e6 60 ]  Winding1="[ 230e3  0.08/30   0.08 ]"  Winding2="[ 25e3  0.08/30  0.08]"  Rm=500  Lm=500  L0=0.5  Saturation="[ 0,0  ;  0.005,1.2  ;  1.0,1.4 ]"  InitialFluxes=[ 0.8 , -0.8 , 0.7 ]  BreakLoop=off  DiscreteSolver=Trapezoidal iterative  DataType=off  TransfoNumber=0
  3500 MW : spsThreePhaseDynamicLoadLib/Three-Phase Dynamic Load  NominalVoltage=[ 25e3 60 ]  ActiveReactivePowers=[3.5e+09 4.44089e-08]  PositiveSequence=[0.991615 -96.3945]  ExternalControl=off  NpNq="[1.5  2.5]"  TimeConstants="[0  0  0  0]"  MinimumVoltage=0.7  Tfilter=1e-4  LoadFlowParameters=[4,0,0,0,0]
      settings: LibrarySourceBlock=|
      | sps_lib/Passives/Three-Phase
      | Dynamic Load
  ASM 575V 5000MVA Pm=4000 MW : spsAsynchronousMachinepuUnitsLib/Asynchronous Machine pu Units  RotorType=Squirrel-cage  PresetModel=No  MechanicalLoad=Torque Tm  ShowDetailedParameters=on  ReferenceFrame=Rotor  Units=pu  MeasurementBus=off  NominalParameters="[5000e6 25e3  60]"  VoltageRatio=1  Stator=[0.01117 0.04832]  Rotor=[0.006 0.04832]  Cage1=[0.01909 0.0397]  Cage2=[0.01909 0.0397]  Lm=2.424  Mechanical="[1  0   2]"  PolePairs=2  InitialConditions=[0.00523668 0 0.941796 0.941796 0.941796 -125.733 -245.733 -5.73298]  SimulateSaturation=off  Saturation="[0.212,0.4201,0.8125,1.0979,1.4799,2.2457,3.2586,4.5763,6.4763 ;   0.5,0.7,0.9,1,1.1,1.2 ,1.3,1.4,1.5]"  LoadFlowParameters=0  TsPowergui=0  TsBlock=-1  IterativeModel=Trapezoidal non iterative  IterativeDiscreteModel=Trapezoidal non iterative  Pmec=4000000000
      settings: LibrarySourceBlock=|
      | sps_lib/Electrical Machines/Asynchronous Machine
      | pu Units
  Load Flow Bus : spsLoadFlowBusLib/Load Flow Bus  LConnTagsString=a  Phases=single  Connectors=on one side  ID=MTL2  Vbase=230e3  Vref=1  Vangle=0  VLF=1.009  VLFb=1  VLFc=1  angleLF=-58.45  angleLFb=0  angleLFc=0
      settings: AttributesFormatString=%<ID>\n%<Vbase>V\n%<VLF>pu\n%<angleLF>deg.
  Load Flow Bus1 : spsLoadFlowBusLib/Load Flow Bus  LConnTagsString=a  Phases=single  Connectors=on one side  ID=MTL_25  Vbase=25e3  Vref=1  Vangle=0  VLF=0.9916  VLFb=1  VLFc=1  angleLF=-96.39  angleLFb=0  angleLFc=0
      settings: AttributesFormatString=%<ID>\n%<Vbase>V\n%<VLF>pu\n%<angleLF>deg.
  MTL 3000 Mvar : spsThreePhaseParallelRLCLoadLib/Three-Phase Parallel RLC Load  LConnTagsString=A|B|C  Configuration=Y (grounded)  NominalVoltage=230e3  Vabc=[1e3 1e3 1e3]  Vabcp=[1e3 1e3 1e3]  NominalFrequency=60  UnbalancedPower=off  ActivePower=0  InductivePower=0  CapacitivePower=3000e6  Pabc=[10e3 9e3 11e3]  QLabc=[100 90 110]  QCabc=[100 90 110]  Pabcp=[10e3 9e3 11e3]  QLabcp=[100 90 110]  QCabcp=[100 90 110]  Measurements=None  LoadType=constant Z
  MTL 4000 MW : spsThreePhaseParallelRLCLoadLib/Three-Phase Parallel RLC Load  LConnTagsString=A|B|C  Configuration=Y (grounded)  NominalVoltage=(25000)*0.991615  Vabc=[1e3 1e3 1e3]  Vabcp=[1e3 1e3 1e3]  NominalFrequency=60  UnbalancedPower=off  ActivePower=4000000000  InductivePower=0  CapacitivePower=0  Pabc=[10e3 9e3 11e3]  QLabc=[100 90 110]  QCabc=[100 90 110]  Pabcp=[10e3 9e3 11e3]  QLabcp=[100 90 110]  QCabcp=[100 90 110]  Measurements=None  LoadType=constant PQ
  MTL 4000 MW1 : spsThreePhaseParallelRLCLoadLib/Three-Phase Parallel RLC Load  LConnTagsString=A|B|C  Configuration=Y (grounded)  NominalVoltage=25e3  Vabc=[1e3 1e3 1e3]  Vabcp=[1e3 1e3 1e3]  NominalFrequency=60  UnbalancedPower=off  ActivePower=4000000000  InductivePower=0  CapacitivePower=0  Pabc=[10e3 9e3 11e3]  QLabc=[100 90 110]  QCabc=[100 90 110]  Pabcp=[10e3 9e3 11e3]  QLabcp=[100 90 110]  QCabcp=[100 90 110]  Measurements=None  LoadType=constant Z
  Terminator_1 : Terminator
  Terminator_2 : Terminator
  Tm : Constant  Value=0.80421
  A : PMIOPort  Side=Left
  B : PMIOPort  Port=2  Side=Left
  C : PMIOPort  Port=3  Side=Left
  wires:
  Tm/1 -> ASM 575V 5000MVA Pm=4000 MW/1
  3500 MW/1 -> Terminator_1/1
  ASM 575V 5000MVA Pm=4000 MW/1 -> Terminator_2/1
  connections:
  A/RConn1 -- 22 000 MVA 735 kV/230 kV/LConn1
  B/RConn1 -- 22 000 MVA 735 kV/230 kV/LConn2
  C/RConn1 -- 22 000 MVA 735 kV/230 kV/LConn3
  230 kV/25 kV 18 000 MVA/LConn1 -- Load Flow Bus/LConn1 -- 22 000 MVA 735 kV/230 kV/RConn1 -- MTL 3000 Mvar/LConn1
  230 kV/25 kV 18 000 MVA/LConn2 -- 22 000 MVA 735 kV/230 kV/RConn2 -- MTL 3000 Mvar/LConn2
  230 kV/25 kV 18 000 MVA/LConn3 -- 22 000 MVA 735 kV/230 kV/RConn3 -- MTL 3000 Mvar/LConn3
  MTL 4000 MW1/LConn1 -- Load Flow Bus1/LConn1 -- MTL 4000 MW/LConn1 -- 230 kV/25 kV 18 000 MVA/RConn1 -- 3500 MW/LConn1 -- ASM 575V 5000MVA Pm=4000 MW/LConn1 -- 1.2  Mvar/LConn1
  MTL 4000 MW1/LConn2 -- MTL 4000 MW/LConn2 -- 230 kV/25 kV 18 000 MVA/RConn2 -- 3500 MW/LConn2 -- ASM 575V 5000MVA Pm=4000 MW/LConn2 -- 1.2  Mvar/LConn2
  230 kV/25 kV 18 000 MVA/RConn3 -- ASM 575V 5000MVA Pm=4000 MW/LConn3 -- 1.2  Mvar/LConn3 -- MTL 4000 MW1/LConn3 -- MTL 4000 MW/LConn3 -- 3500 MW/LConn3
